simulink model "Event6_2018a"  (R2018a)
settings: Solver=FixedStepDiscrete  StartTime=0.0  StopTime=0.1  FixedStep=0.1  RelTol=1e-3  EnableMultiTasking=on
settings Model: Creator=BEAR  LastModifiedBy=apple
settings SolverCC: AutoInsertRateTranBlk=on
settings DataIOCC: LimitDataPoints=on
settings OptimizationCC: LifeSpan=inf
settings DebuggingCC: AllowSymbolicDim=off  SFUnexpectedBacktrackingDiag=warning  SFNoUnconditionalDefaultTransitionDiag=warning  SFExecutionAtInitializationDiag=none
settings CodeAppCC: StateflowObjectComments=on
settings GRTTargetCC: TargetLangStandard=C89/C90 (ANSI)
settings ConfigComp: CovMetricSettings=dw  CovSaveCumulativeToWorkspaceVar=on  CovSaveSingleToWorkspaceVar=on  CovExternalEMLEnable=off  CovSFcnEnable=off

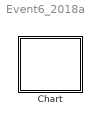
== system Event6_2018a ==
  Chart : Stateflow chart  TreatAsAtomicUnit=on

== stateflow chart Event6_2018a/Chart ==
  state A [parallel]
    settings: executionOrder=1
    state A1
    state A2
    (default) -> A1
    A1 -> A2 : /{E}
  state B [parallel]
    settings: executionOrder=2
    state B1
    state B2
      en: fprintf("en_A2")
    (default) -> B1 : {x=6;}
    B1 -> B2 : E[x>0]{x=x-1;fprintf("a");E}
  data: x local int32
  events: E local FUNCTION_CALL_EVENT
